simulink model "MyPTControlOSM_RTW"  (Simulink 10.1)
settings: Solver=ode1  StartTime=0.0  StopTime=inf  FixedStep=0.0002  RelTol=1e-3
PreLoadFcn:
  | vehicle = 'Car'; if ~length(which('cmcmd')), cmenv; end
  | MyPTControlOSM_RTW_bus
InitFcn:
  | vehicle = 'Car'; if ~length(which('cmcmd')), cmenv; end
  | MyPTControlOSM_RTW_bus
undefined symbols (not defined in the file or in its folder): OperationState, OSMFunc, rv, State
libraries: simulink x14
(part 2 of 2)

== system MyPTControlOSM_RTW/MyPTControlOSM/PowerOn/Wait for PowerOff is ready ==
  Bus In : Inport
  Input : Inport  Port=2
  State 10 Wait for PowerOff is ready : ActionPort  ActionPortLabel=case: { }
  Bus Assignment : BusAssignment  AssignedSignals=State
  Bus Selector : BusSelector  OutputSignals=FuncReturn
  Constant : Constant  Value=11
  Constant1 : Constant  Value=10
  Signal Conversion : SignalConversion  ConversionOutput=Bus copy  OverrideOpt=off
  Switch : Switch  Criteria=u2 ~= 0
  Bus Out : Outport  VectorParamsAs1DForOutWhenUnconnected=off
  wires:
  Signal Conversion/1 -> Bus Out/1
  Bus Assignment/1 -> Signal Conversion/1
  Bus In/1 -> Bus Assignment/1
  Input/1 -> Bus Selector/1
  Bus Selector/1 -> Switch/2  "<FuncReturn>"
  Constant/1 -> Switch/1
  Constant1/1 -> Switch/3
  Switch/1 -> Bus Assignment/2

== system MyPTControlOSM_RTW/MyPTControlOSM/PowerOn/Wait for PowerOn is ready ==
  Bus In : Inport
  Input : Inport  Port=2
  State 7 Wait for PowerOn is ready : ActionPort  ActionPortLabel=case: { }
  Bus Assignment : BusAssignment  AssignedSignals=State
  Bus Selector : BusSelector  OutputSignals=FuncReturn
  Constant : Constant  Value=8
  Constant1 : Constant  Value=7
  Signal Conversion : SignalConversion  ConversionOutput=Bus copy  OverrideOpt=off
  Switch : Switch  Criteria=u2 ~= 0
  Bus Out : Outport  VectorParamsAs1DForOutWhenUnconnected=off
  wires:
  Signal Conversion/1 -> Bus Out/1
  Bus Assignment/1 -> Signal Conversion/1
  Bus In/1 -> Bus Assignment/1
  Input/1 -> Bus Selector/1
  Bus Selector/1 -> Switch/2  "<FuncReturn>"
  Constant/1 -> Switch/1
  Constant1/1 -> Switch/3
  Switch/1 -> Bus Assignment/2

== system MyPTControlOSM_RTW/MyPTControlOSM/PowerOn/Wait for SkipStart is ready ==
  Bus In : Inport
  Input : Inport  Port=2
  State 5 Wait for SkipStart is ready : ActionPort  ActionPortLabel=case: { }
  Bus Assignment : BusAssignment  AssignedSignals=State
  Bus Selector : BusSelector  OutputSignals=FuncReturn
  Constant : Constant  Value=6
  Constant1 : Constant  Value=5
  Signal Conversion : SignalConversion  ConversionOutput=Bus copy  OverrideOpt=off
  Switch : Switch  Criteria=u2 ~= 0
  Bus Out : Outport  VectorParamsAs1DForOutWhenUnconnected=off
  wires:
  Signal Conversion/1 -> Bus Out/1
  Bus Assignment/1 -> Signal Conversion/1
  Bus In/1 -> Bus Assignment/1
  Input/1 -> Bus Selector/1
  Bus Selector/1 -> Switch/2  "<FuncReturn>"
  Constant/1 -> Switch/1
  Constant1/1 -> Switch/3
  Switch/1 -> Bus Assignment/2

== system MyPTControlOSM_RTW/MyPTControlOSM/PowerOn/Wait for Start is ready ==
  Bus In : Inport
  Input : Inport  Port=2
  State 2 Wait for Start is ready : ActionPort  ActionPortLabel=case: { }
  !=KeyPos_KeyIn_Starter : simulink/Logic and Bit Operations/Compare To Constant  SystemSampleTime=-1  relop=~=  const=4  LogicOutDataTypeMode=uint8  ZeroCross=off
  Bus Assignment : BusAssignment  AssignedSignals=State
  Bus Selector : BusSelector  OutputSignals=FuncReturn
  Bus Selector1 : BusSelector  OutputSignals=Key
  Constant : Constant  Value=4
  Constant1 : Constant  Value=2
  Constant2 : Constant  Value=3
  Input Copy : InportShadow  Port=2
  Signal Conversion : SignalConversion  ConversionOutput=Bus copy  OverrideOpt=off
  Skip Start if Key ist not Starter : Switch  Criteria=u2 ~= 0
  Switch : Switch  Criteria=u2 ~= 0
  Bus Out : Outport  VectorParamsAs1DForOutWhenUnconnected=off
  wires:
  Bus Assignment/1 -> Signal Conversion/1
  Signal Conversion/1 -> Bus Out/1
  Bus In/1 -> Bus Assignment/1
  Skip Start if Key ist not Starter/1 -> Switch/3
  Switch/1 -> Bus Assignment/2
  !=KeyPos_KeyIn_Starter/1 -> Skip Start if Key ist not Starter/2
  Constant/1 -> Skip Start if Key ist not Starter/1
  Constant1/1 -> Skip Start if Key ist not Starter/3
  Input Copy/1 -> Bus Selector/1
  Input/1 -> Bus Selector1/1
  Bus Selector1/1 -> !=KeyPos_KeyIn_Starter/1  "<Key>"
  Bus Selector/1 -> Switch/2  "<FuncReturn>"
  Constant2/1 -> Switch/1

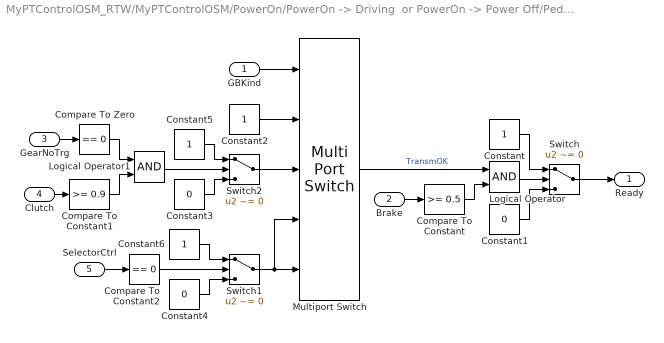
== system MyPTControlOSM_RTW/MyPTControlOSM/PowerOn/PowerOn -> Driving  or PowerOn -> Power Off/PedalsReady2Start ==
  GBKind : Inport
  Brake : Inport  Port=2
  GearNoTrg : Inport  Port=3
  Clutch : Inport  Port=4
  SelectorCtrl : Inport  Port=5
  Compare To Constant : simulink/Logic and Bit Operations/Compare To Constant  SystemSampleTime=-1  relop=>=  const=0.5  LogicOutDataTypeMode=uint8  ZeroCross=off
  Compare To Constant1 : simulink/Logic and Bit Operations/Compare To Constant  SystemSampleTime=-1  relop=>=  const=0.9  LogicOutDataTypeMode=uint8  ZeroCross=off
  Compare To Constant2 : simulink/Logic and Bit Operations/Compare To Constant  SystemSampleTime=-1  relop===  const=0  LogicOutDataTypeMode=uint8  ZeroCross=off
  Compare To Zero : simulink/Logic and Bit Operations/Compare To Zero  SystemSampleTime=-1  relop===  LogicOutDataTypeMode=uint8  ZeroCross=off
  Constant{,2,5..6} (4 alike) : Constant
  Constant1 : Constant  Value=0
  Constant3 : Constant  Value=0
  Constant4 : Constant  Value=0
  Logical Operator : Logic  AllPortsSameDT=off  OutDataTypeStr=boolean
  Logical Operator1 : Logic  AllPortsSameDT=off  OutDataTypeStr=boolean
  Multiport Switch : MultiPortSwitch  DataPortOrder=Zero-based contiguous  Inputs=4  zeroidx=on
  Switch : Switch  Criteria=u2 ~= 0
  Switch1 : Switch  Criteria=u2 ~= 0
  Switch2 : Switch  Criteria=u2 ~= 0
  Ready : Outport  VectorParamsAs1DForOutWhenUnconnected=off
  wires:
  GBKind/1 -> Multiport Switch/1
  Multiport Switch/1 -> Logical Operator/1  "TransmOK"
  Brake/1 -> Compare To Constant/1
  Compare To Constant/1 -> Logical Operator/2
  Switch/1 -> Ready/1
  Logical Operator/1 -> Switch/2
  Constant1/1 -> Switch/3
  Constant/1 -> Switch/1
  Constant2/1 -> Multiport Switch/2
  Switch1/1 -> Multiport Switch/5, Multiport Switch/4
  Switch2/1 -> Multiport Switch/3
  Constant3/1 -> Switch2/3
  Constant4/1 -> Switch1/3
  Constant5/1 -> Switch2/1
  Constant6/1 -> Switch1/1
  Logical Operator1/1 -> Switch2/2
  Clutch/1 -> Compare To Constant1/1
  GearNoTrg/1 -> Compare To Zero/1
  Compare To Zero/1 -> Logical Operator1/1
  Compare To Constant1/1 -> Logical Operator1/2
  SelectorCtrl/1 -> Compare To Constant2/1
  Compare To Constant2/1 -> Switch1/2
